simulink model "one_mass_oscillator"  (R2022b)
settings: Solver=FixedStepAuto  StartTime=0.0  StopTime=120  FixedStep=0.001  RelTol=1e-3
model workspace (MAT data in the model file):
  Amplitude = 5
  J_1 = 1
  d_1 = 1
  k_1 = 10
  omega = 2
settings Model: Creator=yn05ehag  LastModifiedBy=oc47agip
settings SolverCC: AlgebraicLoopSolver=TrustRegion
settings DebuggingCC: UnconnectedInputMsg=warning  UnconnectedOutputMsg=warning  UnconnectedLineMsg=warning  SFMachineParentedDataDiag=warning
settings ModelReferenceCC: EnableRefExpFcnMdlSchedulingChecks=on
settings RTWCC: DLArmComputeVersion=19.05

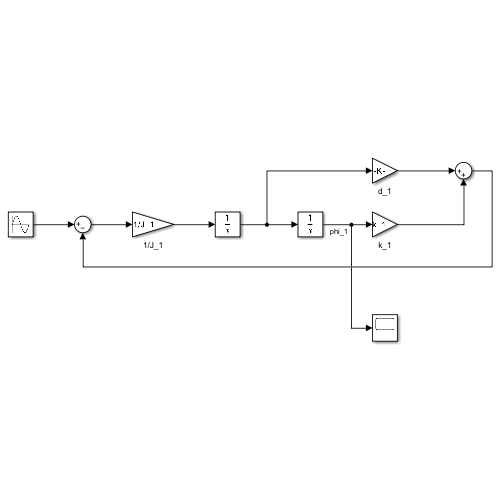
[thumbnail: Simulink's stored preview of the top-level diagram]
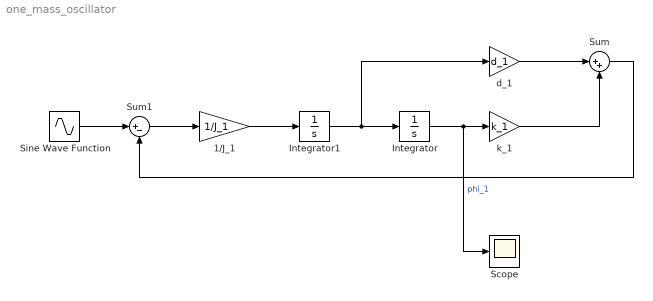
== system one_mass_oscillator ==
  1/J_1 : Gain  Gain=1/J_1
  Integrator : Integrator
  Integrator1 : Integrator
  Scope : Scope
  Sine Wave Function : Sin  Amplitude=Amplitude  Frequency=omega  Phase=pi/2  SampleTime=0
  Sum : Sum  Inputs=|++
  Sum1 : Sum  Inputs=|+-
  d_1 : Gain  Gain=d_1
  k_1 : Gain  Gain=k_1
  wires:
  Integrator1/1 -> d_1/1, Integrator/1
  Integrator/1 -> Scope/1, k_1/1  "phi_1"
  1/J_1/1 -> Integrator1/1
  d_1/1 -> Sum/1
  k_1/1 -> Sum/2
  Sine Wave Function/1 -> Sum1/1
  Sum/1 -> Sum1/2
  Sum1/1 -> 1/J_1/1
